simulink model "lab6"  (R2023b)
settings: Solver=VariableStepAuto  StartTime=0.0  StopTime=5.5  RelTol=1e-3
libraries: spsDCVoltageSourceLib x2, spsDCMachineLib x1, sps_lib x1
settings Model: Creator=Lenovo  LastModifiedBy=Lenovo

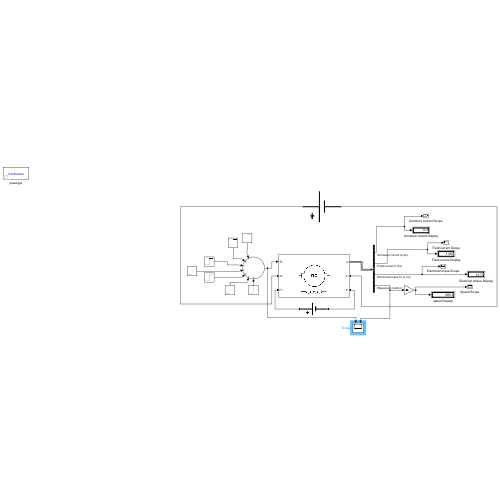
[thumbnail: Simulink's stored preview of the top-level diagram]
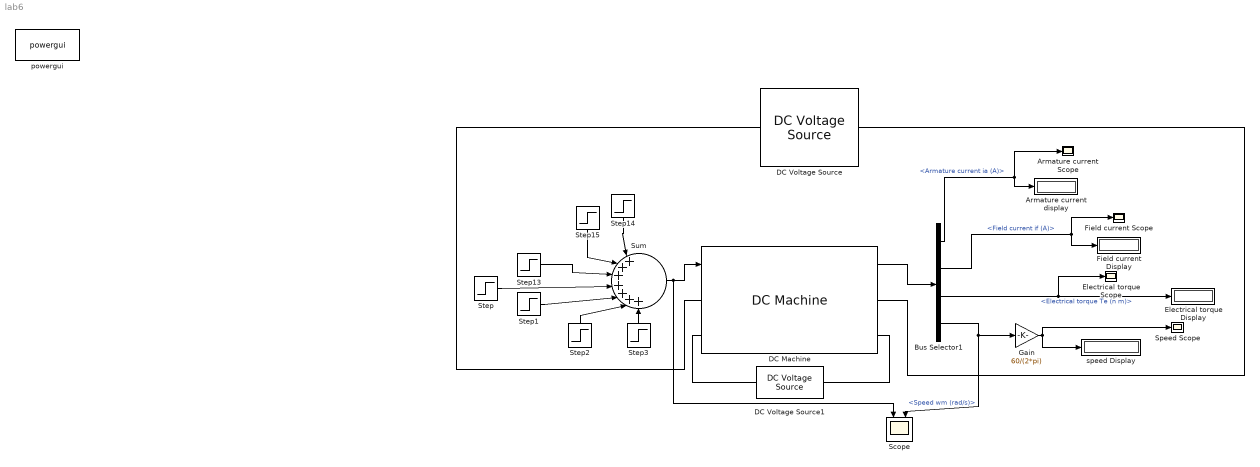
== system lab6 ==
  Armature current Scope : Scope
  Armature current display : Display
  Bus Selector1 : BusSelector  OutputSignals=Armature current ia (A),Field current if (A),Electrical torque Te (n m),Speed wm (rad/s)
  DC Machine : spsDCMachineLib/DC Machine  PresetModel=01: 5HP 240V 1750RPM Field:300V  MechanicalLoad=Torque TL  FieldType=Wound  ShowDetailedParameters=on  MeasurementBus=off  RLa=[2.581 0.028]  RLf=[281.2 156]  Laf=0.9483  MachineConstant=Torque constant (N.m/A)  Ke=1.8  Kt=1.8  J=0.02215  Bm=0.002953  Tf=0.5161  w0=1  Ifinit=1.06685633001422  TsPowergui=0  TsBlock=-1
  DC Voltage Source : spsDCVoltageSourceLib/DC Voltage Source  Amplitude=100  Measurements=None
  DC Voltage Source1 : spsDCVoltageSourceLib/DC Voltage Source  Amplitude=300  Measurements=None
  Electrical torque Display : Display
  Electrical torque Scope : Scope
  Field current Display : Display
  Field current Scope : Scope
  Gain : Gain  Gain=60/(2*pi)
  Scope : Scope  NumInputPorts=2
  Speed Scope : Scope
  Step : Step  Time=4  After=2  SampleTime=0
  Step1 : Step  Time=5  After=2  SampleTime=0
  Step13 : Step  Time=3  After=2  SampleTime=0
  Step14 : Step  After=2  SampleTime=0
  Step15 : Step  Time=2  After=2  SampleTime=0
  Step2 : Step  Time=6  After=2  SampleTime=0
  Step3 : Step  Time=7  After=2  SampleTime=0
  Sum : Sum  Inputs=|+++++++
  powergui : sps_lib/powergui  Priority=1  SimulationMode=Continuous  SampleTime=50e-6  frequency=60  Iterations=50  frequencyindice=0  Pbase=100e6  ErrMax=1e-4  UnitsV=kV  UnitsW=MW  buscounter=0  FunctionMessages=off  echomessages=off  EnableUseOfTLC=off  CurrentSourceSwitches=off  DisableSnubberDevices=off  DisableRonSwitches=off  DisableVfSwitches=off  DisplayEquations=off  AutomaticDiscreteSolvers=off  SolverType=Tustin/Backward Euler (TBE)  Interpol=off  ExternalGateDelay=off  methode=off  Ts=100  x0status=blocks  SPID=on  SwTol=0  HookPort=off  NonlinearTolerance=1e-4  nMaxIteration=100  ContinueOnMaxIteration=off  RestoreLinks=warning  ResistiveCurrentMeasurement=off  Frange=[0:2:500]  Ylog=off  Xlog=on  ShowGrid=off  save=off  variable=ZData  structure=0  ZoomFFT=off  StartTime=0.0  cycles=1  DisplayStyle=1  fundamental=60  FreqAxis=off  MaxFrequency=1000  frequencyindicesteady=1  RmsSteady=1  display=off
  speed Display : Display
  wires:
  Gain/1 -> speed Display/1, Speed Scope/1
  Bus Selector1/1 -> Armature current display/1, Armature current Scope/1  "<Armature current ia (A)>"
  Bus Selector1/2 -> Field current Display/1, Field current Scope/1  "<Field current if (A)>"
  Sum/1 -> DC Machine/1, Scope/1
  Step3/1 -> Sum/7
  Step2/1 -> Sum/6
  Step1/1 -> Sum/5
  Step/1 -> Sum/4
  Step13/1 -> Sum/3
  Step15/1 -> Sum/2
  Step14/1 -> Sum/1
  DC Machine/1 -> Bus Selector1/1
  Bus Selector1/4 -> Gain/1, Scope/2  "<Speed wm (rad/s)>"
  Bus Selector1/3 -> Electrical torque Scope/1, Electrical torque Display/1  "<Electrical torque Te (n m)>"
  connections:
  DC Voltage Source/LConn1 -- DC Machine/RConn1
  DC Voltage Source1/RConn1 -- DC Machine/LConn2
  DC Voltage Source1/LConn1 -- DC Machine/RConn2
  DC Voltage Source/RConn1 -- DC Machine/LConn1
